simulink model "EMPlanner_cs"  (R2021a)
settings: Solver=ode5  StartTime=0.0  StopTime=30  FixedStep=1/1000  RelTol=1e-3
PreLoadFcn:
  | mbxruntime.callbacks.PreLoadFcn(bdroot);
PostLoadFcn:
  | mbxruntime.callbacks.PostLoadFcn(bdroot);
InitFcn:
  | mbxruntime.callbacks.InitFcn(bdroot);
StartFcn:
  | mbxruntime.callbacks.StartFcn(bdroot);
StopFcn:
  | mbxruntime.callbacks.StopFcn(bdroot);
model workspace (MAT data in the model file):
  mbox_table : object (value not decoded)
  model_closed = 0
  sim_status = 0
undefined symbols (not defined in the file or in its folder): aubr, c_factor, cf, cr, DiscIntNeverNeededParam, global_path_x, global_path_y, KD_PID_distance, KD_PID_speed, KI_PID_distance, KI_PID_speed, KP_PID_distance, KP_PID_speed, la, lb, LQR_K1, LQR_K2, LQR_K3, LQR_K4, m, rack_displacement, right_wheel_ground, tablebr, vubr, vx_break_point, warningInitialVelocity, x0
libraries: PreScanSimulinkLibrary x39, simulink x19, simulink_extras x11, Solver_SF x1
(part 9 of 11)

== matlab function EMPlanner_cs/Audi_A8_Sedan_1/decision&planning module/referenceline provider/MATLAB Function6 ==
  data: x_set input; match_point_index_set output; y_set input; frenet_path_x input; frenet_path_y input; frenet_path_heading input; frenet_path_kappa input; proj_x_set output; proj_y_set output; proj_heading_set output; proj_kappa_set output
function [match_point_index_set,proj_x_set, proj_y_set,proj_heading_set,proj_kappa_set] = ...
    fcn(x_set,y_set,frenet_path_x,frenet_path_y,frenet_path_heading,frenet_path_kappa)
%该函数将批量计算x_set，y_set中的xy，在frenet_path下的投影的信息
%输入 x_set,y_set，待投影的点的集合
%x_set,y_set,frenet_path_x,frenet_path_y,frenet_path_heading,frenet_path_kappa
%曲线在直角坐标系下的x，y，heading，kappa
%输出：match_point_index_set 匹配点在frenet_path下的编号的集合(即从全局路径第一个点开始数，第几个点是匹配点)
%     proj_x y heading kappa 投影的x,y,heading,kappa的集合

% 由于事先不知道x_set中到底有多少个点需要投影，因此事先声明一个最大的数量的点作为缓冲
n = 128;
% 并且由于不知道投影点的个数，所以也不知道输出的个数，因此输出也要做缓冲，用nan表示不存在的点
% 输出最多输出128个
% 输出初始化
match_point_index_set = ones(n,1) * nan;
proj_x_set = ones(n,1) * nan;
proj_y_set = ones(n,1) * nan;
proj_heading_set = ones(n,1) * nan;
proj_kappa_set = ones(n,1) * nan;

% 找匹配点，需要利用上一个周期的结果作为下一个周期遍历的起点，因此需要声明两个全局变量

persistent is_first_run;
persistent pre_match_point_index_set;%bug :pre_match_point_index(i) 未必代表的是第i个障碍物的match_point_index
persistent pre_frenet_path_x;
persistent pre_frenet_path_y;
persistent pre_frenet_path_heading;
persistent pre_frenet_path_kappa;
persistent pre_x_set;
persistent pre_y_set;
%算法主函数入口

if isempty(is_first_run)
    %该if分支表示函数首次运行
    is_first_run = 0;
    pre_frenet_path_x = frenet_path_x;
    pre_frenet_path_y = frenet_path_y;
    pre_frenet_path_heading = frenet_path_heading;
    pre_frenet_path_kappa = frenet_path_kappa;
    %要记录首次运行计算的匹配点的结果供下个周期运行，先初始化
    pre_match_point_index_set = ones(n,1) * nan;
    %对x_set,y_set的点做遍历，找到他们的匹配点
    for i = 1 : length(x_set)
        if isnan(x_set(i))
            break;
        end
        %首次运行时，没有任何提示，只能从frenet path的第一个点开始找
        start_search_index = 1;
        % 声明increase_count，用于表示在遍历时distance连续增加的个数
        increase_count = 0;
        % 开始遍历
        min_distance = inf;
        for j = start_search_index : length(frenet_path_x)
            distance = (x_set(i) - frenet_path_x(j))^2 + (y_set(i) - frenet_path_y(j))^2;
            if distance < min_distance
                min_distance = distance;
                match_point_index_set(i) = j;
                increase_count = 0;
            else
                increase_count = increase_count + 1;
            end
            %如果distance连续增加50次就不要再遍历了，节省时间
            if increase_count > 50
                break;
            end
        end
        
        %如何通过匹配点计算投影点，请参见《自动驾驶控制算法第七讲》
        %或《自动驾驶决策规划算法》第一章第三节
        
        %取出匹配点的编号
        match_point_index = match_point_index_set(i);
        %取出匹配点的信息
        match_point_x = frenet_path_x(match_point_index);
        match_point_y = frenet_path_y(match_point_index);
        match_point_heading = frenet_path_heading(match_point_index);
        match_point_kappa = frenet_path_kappa(match_point_index);
        %计算匹配点的方向向量与法向量
        vector_match_point = [match_point_x;match_point_y];
        vector_match_point_direction = [cos(match_point_heading);sin(match_point_heading)];
        %声明待投影点的位矢
        vector_r = [x_set(i);y_set(i)];
        
       %通过匹配点计算投影点
       vector_d = vector_r - vector_match_point;
       ds = vector_d' * vector_match_point_direction;
       vector_proj_point = vector_match_point + ds * vector_match_point_direction;
       proj_heading = match_point_heading + match_point_kappa * ds;
       proj_kappa = match_point_kappa;
       %计算结果输出
       proj_x_set(i) = vector_proj_point(1);
       proj_y_set(i) = vector_proj_point(2);
       proj_heading_set(i) = proj_heading;
       proj_kappa_set(i) = proj_kappa;
    end
    %匹配点的计算结果保存，供下一个周期使用
    pre_match_point_index_set = match_point_index_set;
    pre_x_set = x_set;
    pre_y_set = y_set;
else
    %此if分支表示不是首次运行
    %对每个x_set上的点做处理
    for i = 1 : length(x_set)
        %不是首次运行，对于点x_set(i),y_set(i)来说,start_search_index =
        %pre_match_point_index_set(i)
        start_search_index = pre_match_point_index_set(i);%上个周期匹配点的编号作为本周期搜索的起点
        % 判断帧与帧之间的障碍物是否为同一个
        square_dis = (x_set(i) - pre_x_set(i))^2 + (y_set(i) - pre_y_set(i))^2;
        if square_dis > 36
            % 帧与帧之间的物体的位置距离过大，认为是两个障碍物
            start_search_index = nan;
        end
        % 声明increase_count，用于表示在遍历时distance连续增加的个数
        %%%%%%%%%
        %对于障碍物检测而言，当感知第一次检测到障碍物时，算法并不是首次运行，此时 
        %pre_match_point_index_set的值是nan，如果还用上一时刻的结果作为本周期搜索的起点
        %必然会出问题，所以要修改
        % 声明increase_count_limit
        increase_count_limit = 5;
        if isnan(start_search_index)
            %没有上个周期的结果，那就不能只检查5次了
            increase_count_limit = 50;
            %搜索起点也要设为1
            start_search_index = 1;
        end
        increase_count = 0;
        % 开始遍历
        %这里多一个步骤，判断遍历的方向
        %计算上个周期匹配点的位矢
        vector_pre_match_point = [pre_frenet_path_x(start_search_index);pre_frenet_path_y(start_search_index)];
        vector_pre_match_point_direction = ...
            [cos(pre_frenet_path_heading(start_search_index));sin(pre_frenet_path_heading(start_search_index))];
        %判断遍历的方向
        flag = ([x_set(i);y_set(i)] - vector_pre_match_point)' * vector_pre_match_point_direction;
        min_distance = inf;
        if flag > 0.001
            for j = start_search_index : length(frenet_path_x)
                distance = (x_set(i) - frenet_path_x(j))^2 + (y_set(i) - frenet_path_y(j))^2;
                if distance < min_distance
                    min_distance = distance;
                    match_point_index_set(i) = j;
                    increase_count = 0;
                else
                    increase_count = increase_count + 1;
                end
                %如果distance连续增加increase_count_limit次就不要再遍历了，节省时间
                if increase_count > increase_count_limit
                    break;
                end
            end
        elseif flag < - 0.001
            for j = start_search_index : -1 : 1
                distance = (x_set(i) - frenet_path_x(j))^2 + (y_set(i) - frenet_path_y(j))^2;
                if distance < min_distance
                    min_distance = distance;
                    match_point_index_set(i) = j;
                    increase_count = 0;
                else
                    increase_count = increase_count + 1;
                end
                %如果distance连续增加increase_count_limit次就不要再遍历了，节省时间
                if increase_count > increase_count_limit
                    break;
                end
            end
        else
            match_point_index_set(i) = start_search_index;
        end
        
        %如何通过匹配点计算投影点，请参见《自动驾驶控制算法第七讲》
        %或《自动驾驶决策规划算法》第一章第三节
        
        %取出匹配点的编号
        match_point_index = match_point_index_set(i);
        %取出匹配点的信息
        match_point_x = frenet_path_x(match_point_index);
        match_point_y = frenet_path_y(match_point_index);
        match_point_heading = frenet_path_heading(match_point_index);
        match_point_kappa = frenet_path_kappa(match_point_index);
        %计算匹配点的方向向量与法向量
        vector_match_point = [match_point_x;match_point_y];
        vector_match_point_direction = [cos(match_point_heading);sin(match_point_heading)];
        %声明待投影点的位矢
        vector_r = [x_set(i);y_set(i)];
        
       %通过匹配点计算投影点
       vector_d = vector_r - vector_match_point;
       ds = vector_d' * vector_match_point_direction;
       vector_proj_point = vector_match_point + ds * vector_match_point_direction;
       proj_heading = match_point_heading + match_point_kappa * ds;
       proj_kappa = match_point_kappa;
       %计算结果输出
       proj_x_set(i) = vector_proj_point(1);
       proj_y_set(i) = vector_proj_point(2);
       proj_heading_set(i) = proj_heading;
       proj_kappa_set(i) = proj_kappa;
  
    end
    %匹配点的计算结果保存，供下一个周期使用
    pre_match_point_index_set = match_point_index_set;
    pre_frenet_path_x = frenet_path_x;
    pre_frenet_path_y = frenet_path_y;
    pre_frenet_path_heading = frenet_path_heading;
    pre_frenet_path_kappa = frenet_path_kappa;
    pre_x_set = x_set;
    pre_y_set = y_set;
end

== matlab function EMPlanner_cs/Audi_A8_Sedan_1/decision&planning module/EM Planner/Cartesian2Frenet/MATLAB Function ==
  data: x_set input; s_set output; y_set input; frenet_path_x input; frenet_path_y input; proj_x_set input; proj_y_set input; proj_heading_set input; proj_match_point_index_set input; index2s input; l_set output
function [s_set,l_set] = fcn(x_set,y_set,frenet_path_x,frenet_path_y,...
    proj_x_set,proj_y_set,proj_heading_set,proj_match_point_index_set,index2s)
    %该函数将计算世界坐标系下的x_set，y_set上的点在frenet_path下的坐标s l
    %输入 x_set,y_set 待坐标转换的点
    %     frenet_path_x,frenet_path_y   frenet坐标轴
    %     proj_x,y,heading,kappa,proj_match_point_index 待坐标转换的点的投影点的信息
    %     index2s   frenet_path的index与s的转换表

    % 由于不知道有多少个点需要做坐标转换，所以需要做缓冲
    n = 128;%最多处理128个点
    %输出初始化
    s_set = ones(n,1)*nan;
    l_set = ones(n,1)*nan;
    for i = 1:length(x_set)
        if isnan(x_set(i))
            break;
        end
        %计算s，写个子函数
        s_set(i) = CalcSFromIndex2S(index2s,frenet_path_x,frenet_path_y,proj_x_set(i),proj_y_set(i),...
            proj_match_point_index_set(i));
        n_r = [-sin(proj_heading_set(i));cos(proj_heading_set(i))];
        r_h = [x_set(i);y_set(i)];
        r_r = [proj_x_set(i);proj_y_set(i)];
        l_set(i) = (r_h - r_r)'*n_r;
    end
end

function s = CalcSFromIndex2S(index2s,path_x,path_y,proj_x,proj_y,proj_match_point_index)
  %该函数将计算当指定index2s的映射关系后，计算点proj_x,proj_y的弧长
  vector_1 = [proj_x;proj_y] - [path_x(proj_match_point_index);path_y(proj_match_point_index)];
  %这里要考虑的更全面一些，因为要考虑到proj_match_point_index有可能在path的起点或终点
  if (proj_match_point_index < length(path_x))
      vector_2 = [path_x(proj_match_point_index + 1);path_y(proj_match_point_index + 1)] - ...
          [path_x(proj_match_point_index);path_y(proj_match_point_index)];
  else
      vector_2 = [path_x(proj_match_point_index);path_y(proj_match_point_index)] - ...
          [path_x(proj_match_point_index - 1);path_y(proj_match_point_index - 1)];
  end
  
  if vector_1'*vector_2 > 0
      s = index2s(proj_match_point_index) + sqrt(vector_1'*vector_1);
  else
      s = index2s(proj_match_point_index) - sqrt(vector_1'*vector_1);
  end
  
  
end

== matlab function EMPlanner_cs/Audi_A8_Sedan_1/control module1/control main/chassic steering system/MATLAB Function ==
  data: u input; right_steer output; la input; lb input
function right_steer = fcn(u,la,lb)
if abs(u)<1e-2
   right_steer = u;
else
   R =  (la+lb)/tan(u);
   right_steer = atan((la+lb)/(R+1.624/2));
end

== matlab function EMPlanner_cs/Audi_A8_Sedan_1/control module1/control main/lateral control LQR/calc lqr K ==
  data: k1 input; k output; k2 input; k3 input; k4 input; vx input
function k  = fcn(k1,k2,k3,k4,vx)
    if abs(vx)<0.1
        k=[0,0,0,0];
    else
       
        k=[k1,k2,k3,k4];
    end
end

== matlab function EMPlanner_cs/Audi_A8_Sedan_1/control module1/control main/lateral control LQR/err_kappa_calculate_module ==
  data: x input; y input; phi input; vx input; vy input; phi_dot input; xr input; yr input; thetar input; kappar input; err output; es output; s_dot output; phi output; projection_point_thetar output
function [err,es,s_dot,phi,projection_point_thetar] = fcn(x,y,phi,vx,vy,phi_dot,xr,yr,thetar,kappar)
    
    tor=[cos(thetar);sin(thetar)];
    nor=[-sin(thetar);cos(thetar)];
    d_err=[x-xr;y-yr];
    ed=nor'*d_err;
    es=tor'*d_err;
    %projection_point_thetar=thetar(dmin);%apollo
    projection_point_thetar=thetar+kappar*es;
    ed_dot=vy*cos(phi-projection_point_thetar)+vx*sin(phi-projection_point_thetar);
    %%%%%%%%%
    ephi=sin(phi-projection_point_thetar);
    %%%%%%%%%
    ss_dot=vx*cos(phi-projection_point_thetar)-vy*sin(phi-projection_point_thetar);
    s_dot=ss_dot/(1-kappar*ed);
    ephi_dot=phi_dot-kappar*s_dot;
    err=[ed;ed_dot;ephi;ephi_dot];
    
    
    
    
    
    
    
    
    
    
    
    


end

== matlab function EMPlanner_cs/Audi_A8_Sedan_1/control module1/control main/lateral control LQR/feed_forword_control ==
  data: vx input; a input; forword_angle output; b input; m input; cf input; cr input; k input; kr input
function forword_angle = fcn(vx,a,b,m,cf,cr,k,kr)
    forword_angle=kr*(a+b-b*k(3)-(m*vx*vx/(a+b))*((b/cf)+(a/cr)*k(3)-(a/cr)));
end

== matlab function EMPlanner_cs/Audi_A8_Sedan_1/control module1/control main/lateral control LQR/feedback_control+feedforword_control ==
  data: k input; angle output; err input; forword_angle input
function angle = fcn(k,err,forword_angle)

    angle=-k*err+forword_angle;
end

== matlab function EMPlanner_cs/Audi_A8_Sedan_1/control module1/control main/lateral control LQR/predict_module ==
  data: x input; pred_x_ctrl output; y input; phi input; vx input; vy input; phi_dot input; ts input; pred_y_ctrl output; pred_yaw_ctrl output; pred_vx_ctrl output; pred_vy_ctrl output; pred_yaw_dot_ctrl output
function [pred_x_ctrl,pred_y_ctrl,pred_yaw_ctrl,pred_vx_ctrl,pred_vy_ctrl,pred_yaw_dot_ctrl] = fcn(x,y,phi,vx,vy,phi_dot,ts)
    pred_x_ctrl=x+vx*ts*cos(phi)-vy*ts*sin(phi);
    pred_y_ctrl=y+vy*ts*cos(phi)+vx*ts*sin(phi);
    pred_yaw_ctrl=phi;
    pred_vx_ctrl=vx;
    pred_vy_ctrl=vy;
    pred_yaw_dot_ctrl=phi_dot;
end

== matlab function EMPlanner_cs/Audi_A8_Sedan_1/control module1/control main/longitudinal control double PID/MATLAB Function1 ==
  data: u input; throttle output; brake output
function [throttle,brake] = fcn(u)
    if u>=0
        throttle=u;
        brake=0;
    else
        throttle=0;
        brake=-u;
    end

== matlab function EMPlanner_cs/Audi_A8_Sedan_1/decision&planning module/EM Planner/obs/MATLAB Function2 ==
  data: x_set input; match_point_index_set output; y_set input; frenet_path_x input; frenet_path_y input; frenet_path_heading input; frenet_path_kappa input; proj_x_set output; proj_y_set output; proj_heading_set output; proj_kappa_set output
function [match_point_index_set,proj_x_set, proj_y_set,proj_heading_set,proj_kappa_set] = ...
    fcn(x_set,y_set,frenet_path_x,frenet_path_y,frenet_path_heading,frenet_path_kappa)
%该函数将批量计算x_set，y_set中的xy，在frenet_path下的投影的信息
%输入 x_set,y_set，待投影的点的集合
%x_set,y_set,frenet_path_x,frenet_path_y,frenet_path_heading,frenet_path_kappa
%曲线在直角坐标系下的x，y，heading，kappa
%输出：match_point_index_set 匹配点在frenet_path下的编号的集合(即从全局路径第一个点开始数，第几个点是匹配点)
%     proj_x y heading kappa 投影的x,y,heading,kappa的集合

% 由于事先不知道x_set中到底有多少个点需要投影，因此事先声明一个最大的数量的点作为缓冲
n = 128;
% 并且由于不知道投影点的个数，所以也不知道输出的个数，因此输出也要做缓冲，用nan表示不存在的点
% 输出最多输出128个
% 输出初始化
match_point_index_set = ones(n,1) * nan;
proj_x_set = ones(n,1) * nan;
proj_y_set = ones(n,1) * nan;
proj_heading_set = ones(n,1) * nan;
proj_kappa_set = ones(n,1) * nan;

% 找匹配点，需要利用上一个周期的结果作为下一个周期遍历的起点，因此需要声明两个全局变量

persistent is_first_run;
persistent pre_match_point_index_set;%bug :pre_match_point_index(i) 未必代表的是第i个障碍物的match_point_index
persistent pre_frenet_path_x;
persistent pre_frenet_path_y;
persistent pre_frenet_path_heading;
persistent pre_frenet_path_kappa;
persistent pre_x_set;
persistent pre_y_set;
%算法主函数入口

if isempty(is_first_run)
    %该if分支表示函数首次运行
    is_first_run = 0;
    pre_frenet_path_x = frenet_path_x;
    pre_frenet_path_y = frenet_path_y;
    pre_frenet_path_heading = frenet_path_heading;
    pre_frenet_path_kappa = frenet_path_kappa;
    %要记录首次运行计算的匹配点的结果供下个周期运行，先初始化
    pre_match_point_index_set = ones(n,1) * nan;
    %对x_set,y_set的点做遍历，找到他们的匹配点
    for i = 1 : length(x_set)
        if isnan(x_set(i))
            break;
        end
        %首次运行时，没有任何提示，只能从frenet path的第一个点开始找
        start_search_index = 1;
        % 声明increase_count，用于表示在遍历时distance连续增加的个数
        increase_count = 0;
        % 开始遍历
        min_distance = inf;
        for j = start_search_index : length(frenet_path_x)
            distance = (x_set(i) - frenet_path_x(j))^2 + (y_set(i) - frenet_path_y(j))^2;
            if distance < min_distance
                min_distance = distance;
                match_point_index_set(i) = j;
                increase_count = 0;
            else
                increase_count = increase_count + 1;
            end
            %如果distance连续增加50次就不要再遍历了，节省时间
            if increase_count > 50
                break;
            end
        end
        
        %如何通过匹配点计算投影点，请参见《自动驾驶控制算法第七讲》
        %或《自动驾驶决策规划算法》第一章第三节
        
        %取出匹配点的编号
        match_point_index = match_point_index_set(i);
        %取出匹配点的信息
        match_point_x = frenet_path_x(match_point_index);
        match_point_y = frenet_path_y(match_point_index);
        match_point_heading = frenet_path_heading(match_point_index);
        match_point_kappa = frenet_path_kappa(match_point_index);
        %计算匹配点的方向向量与法向量
        vector_match_point = [match_point_x;match_point_y];
        vector_match_point_direction = [cos(match_point_heading);sin(match_point_heading)];
        %声明待投影点的位矢
        vector_r = [x_set(i);y_set(i)];
        
       %通过匹配点计算投影点
       vector_d = vector_r - vector_match_point;
       ds = vector_d' * vector_match_point_direction;
       vector_proj_point = vector_match_point + ds * vector_match_point_direction;
       proj_heading = match_point_heading + match_point_kappa * ds;
       proj_kappa = match_point_kappa;
       %计算结果输出
       proj_x_set(i) = vector_proj_point(1);
       proj_y_set(i) = vector_proj_point(2);
       proj_heading_set(i) = proj_heading;
       proj_kappa_set(i) = proj_kappa;
    end
    %匹配点的计算结果保存，供下一个周期使用
    pre_match_point_index_set = match_point_index_set;
    pre_x_set = x_set;
    pre_y_set = y_set;
else
    %此if分支表示不是首次运行
    %对每个x_set上的点做处理
    for i = 1 : length(x_set)
        %不是首次运行，对于点x_set(i),y_set(i)来说,start_search_index =
        %pre_match_point_index_set(i)
        start_search_index = pre_match_point_index_set(i);%上个周期匹配点的编号作为本周期搜索的起点
        % 判断帧与帧之间的障碍物是否为同一个
        square_dis = (x_set(i) - pre_x_set(i))^2 + (y_set(i) - pre_y_set(i))^2;
        if square_dis > 36
            % 帧与帧之间的物体的位置距离过大，认为是两个障碍物
            start_search_index = nan;
        end
        % 声明increase_count，用于表示在遍历时distance连续增加的个数
        %%%%%%%%%
        %对于障碍物检测而言，当感知第一次检测到障碍物时，算法并不是首次运行，此时 
        %pre_match_point_index_set的值是nan，如果还用上一时刻的结果作为本周期搜索的起点
        %必然会出问题，所以要修改
        % 声明increase_count_limit
        increase_count_limit = 5;
        if isnan(start_search_index)
            %没有上个周期的结果，那就不能只检查5次了
            increase_count_limit = 50;
            %搜索起点也要设为1
            start_search_index = 1;
        end
        increase_count = 0;
        % 开始遍历
        %这里多一个步骤，判断遍历的方向
        %计算上个周期匹配点的位矢
        vector_pre_match_point = [pre_frenet_path_x(start_search_index);pre_frenet_path_y(start_search_index)];
        vector_pre_match_point_direction = ...
            [cos(pre_frenet_path_heading(start_search_index));sin(pre_frenet_path_heading(start_search_index))];
        %判断遍历的方向
        flag = ([x_set(i);y_set(i)] - vector_pre_match_point)' * vector_pre_match_point_direction;
        min_distance = inf;
        if flag > 0.001
            for j = start_search_index : length(frenet_path_x)
                distance = (x_set(i) - frenet_path_x(j))^2 + (y_set(i) - frenet_path_y(j))^2;
                if distance < min_distance
                    min_distance = distance;
                    match_point_index_set(i) = j;
                    increase_count = 0;
                else
                    increase_count = increase_count + 1;
                end
                %如果distance连续增加increase_count_limit次就不要再遍历了，节省时间
                if increase_count > increase_count_limit
                    break;
                end
            end
        elseif flag < - 0.001
            for j = start_search_index : -1 : 1
                distance = (x_set(i) - frenet_path_x(j))^2 + (y_set(i) - frenet_path_y(j))^2;
                if distance < min_distance
                    min_distance = distance;
                    match_point_index_set(i) = j;
                    increase_count = 0;
                else
                    increase_count = increase_count + 1;
                end
                %如果distance连续增加increase_count_limit次就不要再遍历了，节省时间
                if increase_count > increase_count_limit
                    break;
                end
            end
        else
            match_point_index_set(i) = start_search_index;
        end
        
        %如何通过匹配点计算投影点，请参见《自动驾驶控制算法第七讲》
        %或《自动驾驶决策规划算法》第一章第三节
        
        %取出匹配点的编号
        match_point_index = match_point_index_set(i);
        %取出匹配点的信息
        match_point_x = frenet_path_x(match_point_index);
        match_point_y = frenet_path_y(match_point_index);
        match_point_heading = frenet_path_heading(match_point_index);
        match_point_kappa = frenet_path_kappa(match_point_index);
        %计算匹配点的方向向量与法向量
        vector_match_point = [match_point_x;match_point_y];
        vector_match_point_direction = [cos(match_point_heading);sin(match_point_heading)];
        %声明待投影点的位矢
        vector_r = [x_set(i);y_set(i)];
        
       %通过匹配点计算投影点
       vector_d = vector_r - vector_match_point;
       ds = vector_d' * vector_match_point_direction;
       vector_proj_point = vector_match_point + ds * vector_match_point_direction;
       proj_heading = match_point_heading + match_point_kappa * ds;
       proj_kappa = match_point_kappa;
       %计算结果输出
       proj_x_set(i) = vector_proj_point(1);
       proj_y_set(i) = vector_proj_point(2);
       proj_heading_set(i) = proj_heading;
       proj_kappa_set(i) = proj_kappa;
  
    end
    %匹配点的计算结果保存，供下一个周期使用
    pre_match_point_index_set = match_point_index_set;
    pre_frenet_path_x = frenet_path_x;
    pre_frenet_path_y = frenet_path_y;
    pre_frenet_path_heading = frenet_path_heading;
    pre_frenet_path_kappa = frenet_path_kappa;
    pre_x_set = x_set;
    pre_y_set = y_set;
end

== matlab function EMPlanner_cs/Audi_A8_Sedan_1/decision&planning module/referenceline provider/MATLAB Function3 ==
  data: path_x input; path_heading output; path_y input; path_kappa output
function [path_heading,path_kappa] = fcn(path_x,path_y)
%该函数将计算path的切线方向与x轴的夹角和曲率
%输入：path_x,y路径坐标
%输出：path heading kappa 路径的heading和曲率
%原理 heading = arctan(dy/dx);
%     kappa = dheading/ds;
%     ds = (dx^2 + dy^2)^0.5

%注意，角度的多值性会带来很大的麻烦，需要慎重处理
%例，x 与 x + 2pi往往代表同一个角度，这种多值性在计算曲率会带来麻烦
%比如 原本是(0.1 - (-0.1))/ds，但如果计算出的-0.1多了一个2pi
%kappa就等于(0.1 - (-0.1 + 2*pi))/ds，曲率会变得非常大
%还有若采用中点欧拉法计算heading时，(即使用(y2 - y1)/(x2 - x1)的反正切计算一个角度 ，用(y1 - y0)/(x1
%-x0)的反正切又计算一个角度，然后加起来除以2),如果精确值是 (a1 + a2)/2,但最终计算的结果可能是(a1 + a2 + 2pi)/2
% 还有 tan(x) = tan(x + pi) 所以arctan(tan(x))可能等于x，也可能等于x + pi
% 角度的处理非常麻烦，而且角度处理不当往往是许多奇怪错误的源头

dx = diff(path_x);
dy = diff(path_y);
%用中点欧拉法要比向前欧拉法向后欧拉法更精确，但是也可能计算出的结果比精确值多一个pi
%在这里对dx,dy做中点欧拉法，使用四象限反正切计算角度
dx_pre = [dx(1);dx];
dx_after = [dx;dx(end)];
dx_final = (dx_pre + dx_after)/2;

dy_pre = [dy(1);dy];
dy_after = [dy;dy(end)];
dy_final = (dy_pre + dy_after)/2;

ds_final = sqrt(dx_final.^2 + dy_final.^2);
path_heading = atan2(dy_final,dx_final);

dheading = diff(path_heading);
dheading_pre = [dheading(1);dheading];
dheading_after = [dheading;dheading(end)];
dheading_final = (dheading_pre + dheading_after) / 2;
%为了防止dheading出现多一个2pi的错误，假设真实的dheading较小，用sin(dheading)近似dheading
path_kappa = sin(dheading_final) ./ ds_final;

== matlab function EMPlanner_cs/Audi_A8_Sedan_1/decision&planning module/EM Planner/Cartesian2Frenet/MATLAB Function1 ==
  data: l_set input; s_dot_set output; vx_set input; vy_set input; proj_heading_set input; proj_kappa_set input; l_dot_set output; dl_set output
function [s_dot_set,l_dot_set,dl_set] = fcn(l_set,vx_set,vy_set,proj_heading_set,proj_kappa_set)
%该函数将计算frenet坐标系下的s_dot, l_dot, dl/ds
n = 128;
% 输出初始化
s_dot_set = ones(n,1)*nan;
l_dot_set = ones(n,1)*nan;
dl_set = ones(n,1)*nan;

for i = 1 : length(l_set)
    if isnan(l_set(i))
        break;
    end
    v_h = [vx_set(i);vy_set(i)];
    n_r = [-sin(proj_heading_set(i));cos(proj_heading_set(i))];
    t_r = [cos(proj_heading_set(i));sin(proj_heading_set(i))];
    l_dot_set(i) = v_h'*n_r;
    s_dot_set(i) = v_h'*t_r/(1 - proj_kappa_set(i)*l_set(i));
    %%%向量法做cartesian与frenet的转换要更简单，但是也有缺点，向量法必须依赖速度加速度
    %l' = l_dot/s_dot 但是如果s_dot = 0 此方法就失效了
    if abs(s_dot_set(i)) < 1e-6
        dl_set(i) = 0;
    else
        dl_set(i) = l_dot_set(i)/s_dot_set(i);
    end
end

== matlab function EMPlanner_cs/Audi_A8_Sedan_1/decision&planning module/EM Planner/Cartesian2Frenet/MATLAB Function2 ==
  data: ax_set input; s_dot2_set output; ay_set input; proj_heading_set input; proj_kappa_set input; l_set input; s_dot_set input; dl_set input; l_dot2_set output; ddl_set output
function [s_dot2_set,l_dot2_set,ddl_set] = fcn(ax_set,ay_set,proj_heading_set,proj_kappa_set,l_set,s_dot_set,dl_set)
%由于不知道有多少个点需要做坐标转换，设一个最大值做缓冲
n = 128;
% 输出初始化
s_dot2_set = ones(n,1)*nan;
l_dot2_set = ones(n,1)*nan;
ddl_set = ones(n,1)*nan;

for i = 1:length(l_set)
    if isnan(l_set(i))
       break;
    end
    a_h = [ax_set(i);ay_set(i)];
    n_r = [-sin(proj_heading_set(i));cos(proj_heading_set(i))];
    t_r = [cos(proj_heading_set(i));sin(proj_heading_set(i))];
    %近似认为dkr/ds 为0 简化计算
    l_dot2_set(i) = a_h'*n_r - proj_kappa_set(i) * (1 - proj_kappa_set(i) * l_set(i)) * s_dot_set(i)^2;
    s_dot2_set(i) = (1/(1 - proj_kappa_set(i) * l_set(i)))* (a_h' * t_r + 2 * proj_kappa_set(i) * dl_set(i) * s_dot_set(i)^2);
    % 要考虑加速度为0的情况
    if (s_dot2_set(i) < 1e-6)
        ddl_set(i) = 0;
    else
        ddl_set(i) = (l_dot2_set(i) - dl_set(i)*s_dot2_set(i))/(s_dot_set(i)^2);
    end
end

== matlab function EMPlanner_cs/Audi_A8_Sedan_1/decision&planning module/EM Planner/obs/obs filter ==
  data: host_x input; obs_x_set_final output; host_y input; host_heading_xy input; obs_x_set_gcs input; obs_y_set_gcs input; obs_velocity_set_gcs input; obs_heading_set_gcs input; obs_y_set_final output; obs_velocity_set_final output; obs_heading_set_final output
function [obs_x_set_final,obs_y_set_final,obs_velocity_set_final,obs_heading_set_final] = fcn(host_x,host_y,host_heading_xy,obs_x_set_gcs,obs_y_set_gcs,obs_velocity_set_gcs,obs_heading_set_gcs)
% 该函数将筛选障碍物，纵向[-10,60] 横向[-10,10]的障碍物才会被考虑
% 该函数只是一种单车道的临时办法，考虑到多车道情况，即使障碍物距离较远也应该考虑
% EM Planner完全体是多车道并行计算的，每个车道都生成参考线然后并行计算出多条轨迹，再选择最优的轨迹作为输出

%传感器最多可以识别32个障碍物
n = 32;
%输出初始化
obs_x_set_final = ones(n,1)*nan;
obs_y_set_final = ones(n,1)*nan;
obs_velocity_set_final = ones(n,1)*nan;
obs_heading_set_final = ones(n,1)*nan;
count = 1;
for i = 1:length(obs_x_set_gcs)
    if isnan(obs_x_set_gcs(i))
        break;
    end
    %自车的heading的方向向量与法向量
    tor = [cos(host_heading_xy);sin(host_heading_xy)];
    nor = [-sin(host_heading_xy);cos(host_heading_xy)];
    %障碍物与自车的距离向量
    vector_obs = [obs_x_set_gcs(i);obs_y_set_gcs(i)] - [host_x;host_y];
    %障碍物纵向距离
    lon_distance = vector_obs'*tor;
    %障碍物横向距离
    lat_distance = vector_obs'*nor;
    
    if (lon_distance < 60) && (lon_distance > -10) && (lat_distance > -25) && (lat_distance < 25)
        obs_x_set_final(count) = obs_x_set_gcs(i);
        obs_y_set_final(count) = obs_y_set_gcs(i);
        obs_heading_set_final(count) = obs_heading_set_gcs(i);
        obs_velocity_set_final(count) = obs_velocity_set_gcs(i);
        count = count + 1;
    end
end

== matlab function EMPlanner_cs/Audi_A8_Sedan_1/decision&planning module/EM Planner/MATLAB Function ==
  data: trajectory_heading_final input; y output
function y = fcn(trajectory_heading_final)
y = zeros(421,1);
y(1) = trajectory_heading_final(1);
for i = 2:421
    y(i) = y(i-1) + sin(trajectory_heading_final(i) - trajectory_heading_final(i-1));
end

== matlab function EMPlanner_cs/Audi_A8_Sedan_1/decision&planning module/EM Planner/obs/Cartesian2Frenet1/MATLAB Function ==
  data: x_set input; s_set output; y_set input; frenet_path_x input; frenet_path_y input; proj_x_set input; proj_y_set input; proj_heading_set input; proj_match_point_index_set input; index2s input; l_set output
function [s_set,l_set] = fcn(x_set,y_set,frenet_path_x,frenet_path_y,...
    proj_x_set,proj_y_set,proj_heading_set,proj_match_point_index_set,index2s)
    %该函数将计算世界坐标系下的x_set，y_set上的点在frenet_path下的坐标s l
    %输入 x_set,y_set 待坐标转换的点
    %     frenet_path_x,frenet_path_y   frenet坐标轴
    %     proj_x,y,heading,kappa,proj_match_point_index 待坐标转换的点的投影点的信息
    %     index2s   frenet_path的index与s的转换表

    % 由于不知道有多少个点需要做坐标转换，所以需要做缓冲
    n = 128;%最多处理128个点
    %输出初始化
    s_set = ones(n,1)*nan;
    l_set = ones(n,1)*nan;
    for i = 1:length(x_set)
        if isnan(x_set(i))
            break;
        end
        %计算s，写个子函数
        s_set(i) = CalcSFromIndex2S(index2s,frenet_path_x,frenet_path_y,proj_x_set(i),proj_y_set(i),...
            proj_match_point_index_set(i));
        n_r = [-sin(proj_heading_set(i));cos(proj_heading_set(i))];
        r_h = [x_set(i);y_set(i)];
        r_r = [proj_x_set(i);proj_y_set(i)];
        l_set(i) = (r_h - r_r)'*n_r;
    end
end

function s = CalcSFromIndex2S(index2s,path_x,path_y,proj_x,proj_y,proj_match_point_index)
  %该函数将计算当指定index2s的映射关系后，计算点proj_x,proj_y的弧长
  vector_1 = [proj_x;proj_y] - [path_x(proj_match_point_index);path_y(proj_match_point_index)];
  %这里要考虑的更全面一些，因为要考虑到proj_match_point_index有可能在path的起点或终点
  if (proj_match_point_index < length(path_x))
      vector_2 = [path_x(proj_match_point_index + 1);path_y(proj_match_point_index + 1)] - ...
          [path_x(proj_match_point_index);path_y(proj_match_point_index)];
  else
      vector_2 = [path_x(proj_match_point_index);path_y(proj_match_point_index)] - ...
          [path_x(proj_match_point_index - 1);path_y(proj_match_point_index - 1)];
  end
  
  if vector_1'*vector_2 > 0
      s = index2s(proj_match_point_index) + sqrt(vector_1'*vector_1);
  else
      s = index2s(proj_match_point_index) - sqrt(vector_1'*vector_1);
  end
  
  
end

== matlab function EMPlanner_cs/Audi_A8_Sedan_1/decision&planning module/EM Planner/obs/Cartesian2Frenet1/MATLAB Function1 ==
  data: l_set input; s_dot_set output; vx_set input; vy_set input; proj_heading_set input; proj_kappa_set input; l_dot_set output; dl_set output
function [s_dot_set,l_dot_set,dl_set] = fcn(l_set,vx_set,vy_set,proj_heading_set,proj_kappa_set)
%该函数将计算frenet坐标系下的s_dot, l_dot, dl/ds
n = 128;
% 输出初始化
s_dot_set = ones(n,1)*nan;
l_dot_set = ones(n,1)*nan;
dl_set = ones(n,1)*nan;

for i = 1 : length(l_set)
    if isnan(l_set(i))
        break;
    end
    v_h = [vx_set(i);vy_set(i)];
    n_r = [-sin(proj_heading_set(i));cos(proj_heading_set(i))];
    t_r = [cos(proj_heading_set(i));sin(proj_heading_set(i))];
    l_dot_set(i) = v_h'*n_r;
    s_dot_set(i) = v_h'*t_r/(1 - proj_kappa_set(i)*l_set(i));
    %%%向量法做cartesian与frenet的转换要更简单，但是也有缺点，向量法必须依赖速度加速度
    %l' = l_dot/s_dot 但是如果s_dot = 0 此方法就失效了
    if abs(s_dot_set(i)) < 1e-6
        dl_set(i) = 0;
    else
        dl_set(i) = l_dot_set(i)/s_dot_set(i);
    end
end

== matlab function EMPlanner_cs/Audi_A8_Sedan_2/PathFollower_Preview_1/LateralController/CTRL REFERENCES/Calculate Lateral Error/eml_find_10k_lateral_error_points ==
  data: pvp input size=2; dist_psvehicle output size=10; TrajOffset_x_y_Y input size=3; ActorOffset_Left_Right input; p0 input size=2; PreviewDistance input size=10; Traj_x parameter; Traj_y parameter; Traj_t parameter; Traj_v parameter; RefreshCounter parameter
function dist_psvehicle  = eml_find_10k_lateral_error_points(pvp,TrajOffset_x_y_Y,ActorOffset_Left_Right,p0,PreviewDistance,Traj_x,Traj_y,Traj_t,Traj_v,RefreshCounter)

dist_psvehicle = emlfcn_find_10k_lateral_error_points(pvp,TrajOffset_x_y_Y,ActorOffset_Left_Right,p0,PreviewDistance,Traj_x,Traj_y,Traj_t,Traj_v,RefreshCounter);

% end function

== matlab function EMPlanner_cs/Audi_A8_Sedan_1/decision&planning module/EM Planner/obs/Cartesian2Frenet1/MATLAB Function2 ==
  data: ax_set input; s_dot2_set output; ay_set input; proj_heading_set input; proj_kappa_set input; l_set input; s_dot_set input; dl_set input; l_dot2_set output; ddl_set output
function [s_dot2_set,l_dot2_set,ddl_set] = fcn(ax_set,ay_set,proj_heading_set,proj_kappa_set,l_set,s_dot_set,dl_set)
%由于不知道有多少个点需要做坐标转换，设一个最大值做缓冲
n = 128;
% 输出初始化
s_dot2_set = ones(n,1)*nan;
l_dot2_set = ones(n,1)*nan;
ddl_set = ones(n,1)*nan;

for i = 1:length(l_set)
    if isnan(l_set(i))
       break;
    end
    a_h = [ax_set(i);ay_set(i)];
    n_r = [-sin(proj_heading_set(i));cos(proj_heading_set(i))];
    t_r = [cos(proj_heading_set(i));sin(proj_heading_set(i)];
    %近似认为dkr/ds 为0 简化计算
    l_dot2_set(i) = a_h'*n_r - proj_kappa_set(i) * (1 - proj_kappa_set(i) * l_set(i)) * s_dot_set(i)^2;
    s_dot2_set(i) = (1/(1 - proj_kappa_set(i) * l_set(i)))* (a_h' * t_r + 2 * proj_kappa_set(i) * dl_set(i) * s_dot_set(i)^2);
    % 要考虑加速度为0的情况
    if (s_dot2_set(i) < 1e-6)
        ddl_set(i) = 0;
    else
        ddl_set(i) = (l_dot2_set(i) - dl_set(i)*s_dot2_set(i))/(s_dot_set(i)^2);
    end
end

== matlab function EMPlanner_cs/Audi_A8_Sedan_1/decision&planning module/EM Planner/obs/MATLAB Function ==
  data: obs_x_set_gcs input; static_obs_x_set output; obs_y_set_gcs input; obs_heading_set_gcs input; obs_velocity_set_gcs input; static_obs_y_set output; dynamic_obs_x_set output; dynamic_obs_y_set output; dynamic_obs_vx_set output; dynamic_obs_vy_set output
function [static_obs_x_set,static_obs_y_set,dynamic_obs_x_set,dynamic_obs_y_set,dynamic_obs_vx_set,dynamic_obs_vy_set]...
    = fcn(obs_x_set_gcs,obs_y_set_gcs,obs_heading_set_gcs,obs_velocity_set_gcs)

%该函数将分类静态障碍物和动态障碍物
%输出初始化
n = 32;
static_obs_x_set = ones(n,1)*nan;
static_obs_y_set = ones(n,1)*nan;
dynamic_obs_x_set = ones(n,1)*nan;
dynamic_obs_y_set = ones(n,1)*nan;
dynamic_obs_vx_set = ones(n,1)*nan;
dynamic_obs_vy_set = ones(n,1)*nan;
count_static = 1;
count_dynamic = 1;
for i = 1:length(obs_x_set_gcs)
    if isnan(obs_velocity_set_gcs(i))
        break;
    end
    if abs(obs_velocity_set_gcs(i)) < 0.1
        static_obs_x_set(count_static) = obs_x_set_gcs(i);
        static_obs_y_set(count_static) = obs_y_set_gcs(i);
        count_static = count_static + 1;
    else
        dynamic_obs_x_set(count_dynamic) = obs_x_set_gcs(i);
        dynamic_obs_y_set(count_dynamic) = obs_y_set_gcs(i);
        dynamic_obs_vx_set(count_dynamic) = obs_velocity_set_gcs(i)*cos(obs_heading_set_gcs(i));
        dynamic_obs_vy_set(count_dynamic) = obs_velocity_set_gcs(i)*sin(obs_heading_set_gcs(i));
        count_dynamic = count_dynamic + 1;      
    end
end

== matlab function EMPlanner_cs/Audi_A8_Sedan_1/decision&planning module/EM Planner/calc path length and map between point and s ==
  data: trajectory_x input; path_s_end output; trajectory_y input; path_index2s output
function [path_s_end,path_index2s] = fcn(trajectory_x,trajectory_y)
% 该函数将计算以trajectory的s 与 x y 的对应关系，可以看作是trajectory index2s
n = length(trajectory_x);
path_index2s = zeros(n,1);
sum = 0;
for i = 2:length(trajectory_x)
    if isnan(trajectory_x(i))
        break;
    end
    sum = sum + sqrt((trajectory_x(i) - trajectory_x(i-1))^2 + (trajectory_y(i) - trajectory_y(i-1))^2);
    path_index2s(i) = sum;
end
% 计算出trajectory的长度
if i == n
    path_s_end = path_index2s(end);
else
    % 因为循环的退出条件为isnan(trajectory_x(i)) 所以 i 所对应的数为 nan 
    path_s_end = path_index2s(i - 1);
end

== matlab function EMPlanner_cs/Audi_A8_Sedan_1/decision&planning module/EM Planner/path decision task/increase DP path nodes ==
  data: dp_path_s_init input; dp_path_s_final output; dp_path_l_init input; plan_start_s input; plan_start_l input; plan_start_dl input; plan_start_ddl input; dp_path_l_final output; dp_path_dl_final output; dp_path_ddl_final output
function [dp_path_s_final,dp_path_l_final,dp_path_dl_final,dp_path_ddl_final] = ...
    fcn(dp_path_s_init,dp_path_l_init,plan_start_s,plan_start_l,plan_start_dl,plan_start_ddl)
% 该函数将增密dp_path_s,dp_path_l
% 由于事先不知道动态规划采样的行和列，也就不知道动态规划计算的曲线有多长，因此需要做缓冲
% 每1“米”采样一个点，一共采60个
ds = 1;
% 输出初始化
dp_path_s_final = ones(60,1)*nan;
dp_path_l_final = ones(60,1)*nan;
dp_path_dl_final = ones(60,1)*nan;
dp_path_ddl_final = ones(60,1)*nan;

% 设置五次多项式的起点
start_s = plan_start_s;
start_l = plan_start_l;
start_dl = plan_start_dl;
start_ddl = plan_start_ddl;

s_cur = [];
l_temp = [];
dl_temp =[];
ddl_temp = [];

for i = 1:length(dp_path_s_init)
    if dp_path_s_init(i) == -1
        break;
    end
    for j = 1:10000
        %采样s
        s_node = start_s + ds*(j - 1);
        if s_node < dp_path_s_init(i)
            s_cur = [s_cur,s_node];
        else
            break;
        end
    end
    end_s = dp_path_s_init(i);
    end_l = dp_path_l_init(i);
    end_dl = 0;
    end_ddl = 0;
    coeff = CalcQuinticCoeffient(start_l,start_dl,start_ddl,end_l,end_dl,end_ddl,start_s,end_s);
    a0 = coeff(1);
    a1 = coeff(2);
    a2 = coeff(3);
    a3 = coeff(4);
    a4 = coeff(5);
    a5 = coeff(6);
    l = a0 * ones(1,length(s_cur)) + a1 * s_cur + a2 * s_cur.^2 + a3 * s_cur.^3 +...
        a4 * s_cur.^4 + a5 * s_cur.^5;
    dl = a1 * ones(1,length(s_cur)) + 2 * a2 * s_cur + 3 * a3 * s_cur.^2 + ...
        4 * a4 * s_cur.^3 + 5 * a5 * s_cur.^4;
    ddl = 2 * a2 * ones(1,length(s_cur)) + 6 * a3 * s_cur + 12 * a4 * s_cur.^2 + ...
        20 * a5 * s_cur.^3;
    % 把 l dl ddl 的结果保存
    l_temp = [l_temp,l];
    dl_temp = [dl_temp,dl];
    ddl_temp = [ddl_temp,ddl];
    % end的值赋值给start 做下一步循环
    start_s = end_s;
    start_l = end_l;
    start_dl = end_dl;
    start_ddl = end_ddl;
    s_cur = [];
end
   for k = 1:length(l_temp)
       if k == 61
           break;
       end
       dp_path_s_final(k) = plan_start_s + ds * (k - 1);
       dp_path_l_final(k) = l_temp(k);
       dp_path_dl_final(k) = dl_temp(k);
       dp_path_ddl_final(k) = ddl_temp(k);
   end
end

function coeff = CalcQuinticCoeffient(start_l,start_dl,start_ddl,end_l,end_dl,end_ddl,start_s,end_s)
    % l = a0 + a1*s + a2*s^2 + a3*s^3 + a4*s^4 + a5*s^5
    % l' = a1 + 2 * a2 * s + 3 * a3 * s^2 + 4 * a4 * s^3 + 5 * a5 * s^4
    % l'' = 2 * a2 + 6 * a3 * s + 12 * a4 * s^2 + 20 * a5 * s^3
    start_s2 = start_s * start_s;
    start_s3 = start_s2 * start_s;
    start_s4 = start_s3 * start_s;
    start_s5 = start_s4 * start_s;
    end_s2 = end_s * end_s;
    end_s3 = end_s2 * end_s;
    end_s4 = end_s3 * end_s;
    end_s5 = end_s4 * end_s;
    A = [1,start_s, start_s2,     start_s3,     start_s4,      start_s5;
         0 1,       2 * start_s,  3 * start_s2, 4 * start_s3,  5 * start_s4;
         0 0,       2,            6 * start_s,  12 * start_s2, 20 * start_s3;
         1,end_s, end_s2,     end_s3,     end_s4,      end_s5;
         0,1,     2 * end_s,  3 * end_s2, 4 * end_s3,  5 * end_s4;
         0,0,     2,          6 * end_s,  12 * end_s2, 20 * end_s3;];
    B = [start_l;
         start_dl;
         start_ddl;
         end_l;
         end_dl;
         end_ddl;];
     coeff = A \ B;
    
end

== matlab function EMPlanner_cs/Audi_A8_Sedan_1/decision&planning module/EM Planner/Frenet2Cartesian task ==
  data: s_set input; x_set output; l_set input; dl_set input; ddl_set input; frenet_path_x input; frenet_path_y input; frenet_path_heading input; frenet_path_kappa input; index2s input; y_set output; heading_set output; kappa_set output
function [x_set,y_set,heading_set,kappa_set] = ...
    fcn(s_set,l_set,dl_set,ddl_set,frenet_path_x,frenet_path_y,frenet_path_heading,frenet_path_kappa,index2s)
% 通用算法 frenet转frenet
% 由于不知道有多少个(s,l)要转化成直角坐标，因此做缓冲
% 输出初始化
    x_set = ones(600,1) * nan;
    y_set = ones(600,1) * nan;
    heading_set = ones(600,1) * nan;
    kappa_set = ones(600,1) * nan;
    for i = 1:length(s_set)
        if isnan(s_set(i))
            break;
        end
        % 计算(s,l)在frenet坐标轴上的投影
        [proj_x,proj_y,proj_heading,proj_kappa] = CalcProjPoint(s_set(i),frenet_path_x,frenet_path_y,frenet_path_heading,...
    frenet_path_kappa,index2s);
        nor = [-sin(proj_heading);cos(proj_heading)];
        point = [proj_x;proj_y] + l_set(i) * nor;
        x_set(i) = point(1);
        y_set(i) = point(2);
        heading_set(i) = proj_heading + atan(dl_set(i)/(1 - proj_kappa * l_set(i)));
        % 近似认为 kappa' == 0,frenet转cartesian公式，见第一章第三节评论区的链接
        kappa_set(i) = ((ddl_set(i) + proj_kappa * dl_set(i) * tan(heading_set(i) - proj_heading)) * ...
            (cos(heading_set(i) - proj_heading)^2)/(1 - proj_kappa * l_set(i)) + proj_kappa) * ...
            cos(heading_set(i) - proj_heading)/(1 - proj_kappa * l_set(i));
         
    end

end


function [proj_x,proj_y,proj_heading,proj_kappa] = CalcProjPoint(s,frenet_path_x,frenet_path_y,frenet_path_heading,...
    frenet_path_kappa,index2s)
% 该函数将计算在frenet坐标系下，点(s,l)在frenet坐标轴的投影的直角坐标(proj_x,proj_y,proj_heading,proj_kappa)'
% 先找匹配点的编号
    match_index = 1;
    while index2s(match_index) < s
        match_index = match_index + 1;
    end
    match_point = [frenet_path_x(match_index);frenet_path_y(match_index)];
    match_point_heading = frenet_path_heading(match_index);
    match_point_kappa = frenet_path_kappa(match_index);
    ds = s - index2s(match_index);
    match_tor = [cos(match_point_heading);sin(match_point_heading)];
    proj_point = match_point + ds * match_tor;
    proj_heading = match_point_heading + ds * match_point_kappa;
    proj_kappa = match_point_kappa;
    proj_x = proj_point(1);
    proj_y = proj_point(2);   
end

== matlab function EMPlanner_cs/Audi_A8_Sedan_1/decision&planning module/EM Planner/path and speed merge ==
  data: s input; trajectory_x output; s_dot input; s_dot2 input; relative_time input; current_time input; path_s input; trajectory_x_init input; trajectory_y_init input; trajectory_heading_init input; trajectory_kappa_init input; trajectory_y output; trajectory_heading output; trajectory_kappa output; trajectory_speed output; trajectory_accel output; trajectory_time output
function [trajectory_x,trajectory_y,trajectory_heading,trajectory_kappa,trajectory_speed,trajectory_accel,trajectory_time] = ...
    fcn(s,s_dot,s_dot2,relative_time,current_time,path_s,trajectory_x_init,trajectory_y_init,trajectory_heading_init,trajectory_kappa_init)
% 该函数将合并path和speed
% 由于path 是 60个点，speed 有 401个点，合并后，path和speed有401个点，因此需要做插值
n = 401;
trajectory_x = zeros(n,1);
trajectory_y = zeros(n,1);
trajectory_heading = zeros(n,1);
trajectory_kappa = zeros(n,1);
trajectory_speed = zeros(n,1);

trajectory_accel = zeros(n,1);
index = 1;
% 由于trajectory_x_init中不是所有的值都有效，(有nan) 所以要找到有效值的范围
while ~isnan(trajectory_x_init(index)) 
    index = index + 1;
end
index = index - 1;
trajectory_time = zeros(n,1);
for i = 1:n-1
    %interp1 线性插值
    % 若 x = [1,2] y = [3,4]
    %interp1(x,y,1.5) 会得到3.5
    %interp1 的缺点是 在端点或超过端点的，结果为nan
    % interp1(x,y,2) 不会等于4 而是会等于nan
    % interp1(x,y,6) 也会等于nan，所以在端点处要单独处理
    trajectory_x(i) = interp1(path_s(1:index),trajectory_x_init(1:index),s(i));
    trajectory_y(i) = interp1(path_s(1:index),trajectory_y_init(1:index),s(i));
    trajectory_heading(i) = interp1(path_s(1:index),trajectory_heading_init(1:index),s(i));
    trajectory_kappa(i) = interp1(path_s(1:index),trajectory_kappa_init(1:index),s(i));
    trajectory_time(i) = relative_time(i) + current_time;%速度规划会得到相对时间，转换成绝对时间
    trajectory_speed(i) = s_dot(i);
    trajectory_accel(i) = s_dot2(i);
end
% 端点单独处理
trajectory_x(end) = trajectory_x_init(end);
trajectory_y(end) = trajectory_y_init(end);
trajectory_heading(end) = trajectory_heading_init(end);
trajectory_kappa(end) = trajectory_kappa_init(end);
trajectory_time(end) = relative_time(end) + current_time;
trajectory_speed(end) = s_dot(end);
trajectory_accel(end) = s_dot2(end);

== matlab function EMPlanner_cs/Audi_A8_Sedan_1/decision&planning module/EM Planner/increase st point count ==
  data: s_init input; s output; s_dot_init input; s_dot2_init input; relative_time_init input; s_dot output; s_dot2 output; relative_time output
function [s,s_dot,s_dot2,relative_time] = fcn(s_init,s_dot_init,s_dot2_init,relative_time_init)
%该函数将增密s s_dot s_dot2
% 为什么需要增密，因为控制的执行频率是规划的10倍，轨迹点如果不够密，必然会导致规划效果不好
% 但是若在速度二次规划中点取的太多，会导致二次规划的矩阵规模太大计算太慢
% 所以方法是在二次规划中选取少量的点优化完毕后，在用此函数增密
t_end = length(relative_time_init);
for i = 1:length(relative_time_init)
    if isnan(relative_time_init(i))
        t_end = i - 1;
        break;
    end
end
T = relative_time_init(t_end);
n = 401;
dt = T/(n-1);
s = zeros(n,1);
s_dot = zeros(n,1);
s_dot2 = zeros(n,1);
relative_time = zeros(n,1);
for i = 1:n
    current_t = (i-1)*dt;
    for j = 1:t_end - 1
        if relative_time_init(j) <= current_t && relative_time_init(j+1) > current_t
            break;
        end
    end
    x = current_t - relative_time_init(j);
    s(i) = s_init(j) + s_dot_init(j)*x + (1/3)*s_dot2_init(j)*x^2 + (1/6)*s_dot2_init(j+1)*x^2; 
    s_dot(i) = s_dot_init(j) + 0.5*s_dot2_init(j)*x + 0.5*s_dot2_init(j+1)*x;
    s_dot2(i) = s_dot2_init(j) + (s_dot2_init(j+1) - s_dot2_init(j))*x/(relative_time_init(j+1) - relative_time_init(j));
    relative_time(i) = current_t;
end

== matlab function EMPlanner_cs/Audi_A8_Sedan_1/control module1/MATLAB Function ==
  data: trajectory_x input; xr output; trajectory_y input; trajectory_heading input; trajectory_kappa input; trajectory_speed input; trajectory_accel input; trajectory_time input; current_time input; yr output; thetar output; kappar output; vr output; ar output
function [xr,yr,thetar,kappar,vr,ar] = fcn(trajectory_x,trajectory_y,trajectory_heading,...
    trajectory_kappa,trajectory_speed,trajectory_accel,trajectory_time,current_time)
% 该函数根据规划的轨迹计算出期望跟踪的点
% 由于控制也是有延迟，所以控制发出的期望跟踪的点是current_time + 0.01;
control_time = current_time + 0.01;
% 规划发出的轨迹有一部分是拼接的，在刚启动的时候，stitch_time = -1,因此要先把它去掉
start_index = 1;
while (trajectory_time(start_index) == -1)
    start_index = start_index + 1;
end
% 使用interp1插值计算得到xr yr thetar,kappar,vr,ar
% 由于interp1在端点会得到nan，因此需要防一手
% 解释，为什么需要trajectory_time(start_index) ~= 0
% 因为在刚启动时规划先执行(100ms)，当规划完毕的时候控制已经执行了10次
% 那么在最开始的时候，规划还没给结果是控制已经执行了10次，在这10次中控制跟踪的轨迹是空轨迹
% simulink 空轨迹表示为 0，0，0，0，0，0......,这样trajectory_time
% 也全是0，trajectory_time不单调递增
% 而interp1(x,y,x0)要求x必须要单调递增，否则会报错，所以当规划首次运行时控制需要执行下面这个else分支的代码，否则会报错
if control_time > trajectory_time(start_index) && trajectory_time(start_index) ~= 0
    xr = interp1(trajectory_time(start_index:end),trajectory_x(start_index:end),control_time);
    yr = interp1(trajectory_time(start_index:end),trajectory_y(start_index:end),control_time);
    thetar = interp1(trajectory_time(start_index:end),trajectory_heading(start_index:end),control_time);
    kappar = interp1(trajectory_time(start_index:end),trajectory_kappa(start_index:end),control_time);
    vr = interp1(trajectory_time(start_index:end),trajectory_speed(start_index:end),control_time);
    ar = interp1(trajectory_time(start_index:end),trajectory_accel(start_index:end),control_time);
else
    xr = trajectory_x(start_index);
    yr = trajectory_y(start_index);
    thetar = trajectory_heading(start_index);
    kappar = trajectory_kappa(start_index);
    vr = trajectory_speed(start_index);
    ar = trajectory_accel(start_index);
end

== matlab function EMPlanner_cs/Audi_A8_Sedan_1/decision&planning module/EM Planner/stitch trajectory ==
  data: trajectory_x input; trajectory_x_final output; trajectory_y input; trajectory_heading input; trajectory_kappa input; trajectory_speed input; trajectory_accel input; trajectory_time input; stitch_x input; stitch_y input; stitch_heading input; stitch_kappa input; stitch_speed input; stitch_accel input; stitch_time input; trajectory_y_final output; trajectory_heading_final output; trajectory_kappa_final output; trajectory_speed_final output; trajectory_accel_final output; trajectory_time_final output
function [trajectory_x_final,trajectory_y_final,trajectory_heading_final,trajectory_kappa_final,...
          trajectory_speed_final,trajectory_accel_final,trajectory_time_final] = fcn(trajectory_x,...
          trajectory_y,trajectory_heading,trajectory_kappa,trajectory_speed,trajectory_accel,trajectory_time,...
          stitch_x,stitch_y,stitch_heading,stitch_kappa,stitch_speed,stitch_accel,stitch_time)
% 轨迹拼接，把stitch trajectory 拼到规划完成的轨迹上
n = 401 + 20;
trajectory_x_final = zeros(n,1);
trajectory_y_final = zeros(n,1);
trajectory_heading_final = zeros(n,1);
trajectory_kappa_final = zeros(n,1);
trajectory_speed_final = zeros(n,1);
trajectory_accel_final = zeros(n,1);
trajectory_time_final = zeros(n,1);

trajectory_x_final = [stitch_x;trajectory_x];
trajectory_y_final = [stitch_y;trajectory_y];
trajectory_heading_final = [stitch_heading;trajectory_heading];
trajectory_kappa_final = [stitch_kappa;trajectory_kappa];
trajectory_speed_final = [stitch_speed;trajectory_speed];
trajectory_accel_final = [stitch_accel;trajectory_accel];
trajectory_time_final = [stitch_time;trajectory_time];
